simulink model "traslacion_carro"  (R2019a)
settings: Solver=VariableStepAuto  StartTime=0.0  StopTime=10.0  RelTol=1e-3
values from neighbouring files (symbols this model uses):
  b_t = 90.0    (= 90)    [parametros.m]
  b_tb = 5.0e6    (= 5000000)    [parametros.m]
  b_td_eq = ( b_td + i_t^2*b_tm ) / (r_td^2)    (= 21607.2)    [parametros.m]
  b_tw = 3.0e3    (= 3000)    [parametros.m]
  i_t = 30.0    (= 30)    [parametros.m]
  K_tw = 4.8e5    (= 480000)    [parametros.m]
  M_t = 30000    [parametros.m]
  m_td_eq = ( J_td + i_t^2*J_tm_tb ) / (r_td^2)    (= 30000)    [parametros.m]
  r_td = 0.50    (= 0.5)    [parametros.m]
  T_tb_max = 5.0e3    (= 5000)    [parametros.m]
  x_t0 = -30.0    (= -30)    [parametros.m]
  x_td0 = x_t0    (= -30)    [parametros.m]
settings Model: Creator=Facundo  LastModifiedBy=Facundo
settings DataIOCC: SaveOutput=off  SaveTime=off

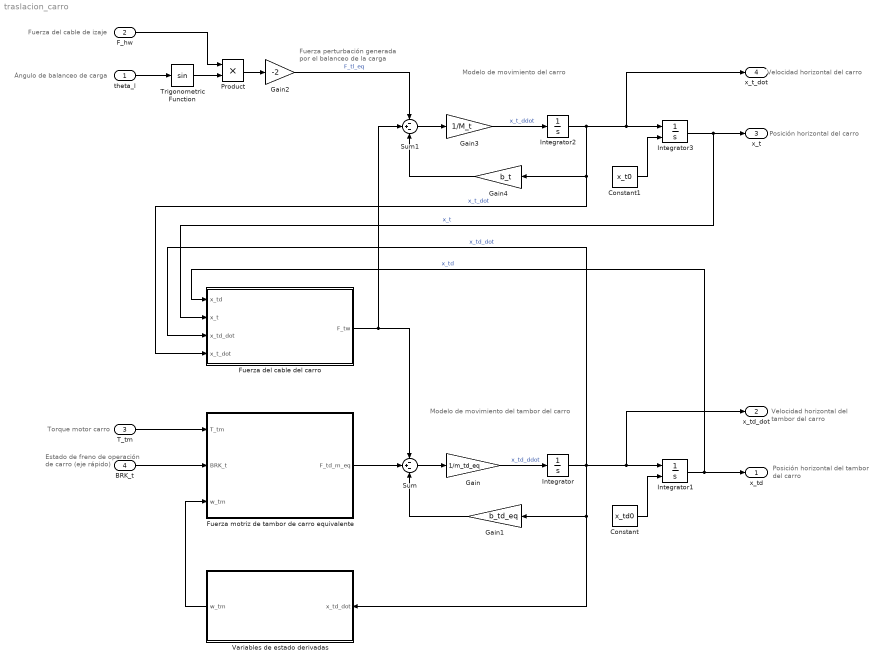
== system traslacion_carro ==
  note: Velocidad horizontal
      | del tambor del carro
  note: Velocidad horizontal del carro
  note: Modelo de movimiento del carro
  note: Fuerza perturbación generada
      | por el balanceo de la carga
  note: Posición horizontal del carro
  note: Estado de freno de
      | operación de carro
      | (eje rápido)
  note: Torque motor carro
  note: Modelo de movimiento del tambor del carro
  note: Fuerza del cable de izaje
  note: Ángulo de balanceo de carga
  note: Posición horizontal
      | del tambor del carro
  theta_l : Inport  OutDataTypeStr=double  PortDimensions=1  SampleTime=0
  F_hw : Inport  Port=2  OutDataTypeStr=double  PortDimensions=1  SampleTime=0
  T_tm : Inport  Port=3
  BRK_t : Inport  Port=4
  Constant : Constant  Value=x_td0
  Constant1 : Constant  Value=x_t0
  Fuerza del cable del carro : Subsystem
  Fuerza motriz de tambor de carro equivalente : Subsystem
  Gain : Gain  Gain=1/m_td_eq
  Gain1 : Gain  Gain=b_td_eq
  Gain2 : Gain  Gain=-2
  Gain3 : Gain  Gain=1/M_t
  Gain4 : Gain  Gain=b_t
  Integrator : Integrator
  Integrator1 : Integrator  InitialConditionSource=external
  Integrator2 : Integrator
  Integrator3 : Integrator  InitialConditionSource=external
  Product : Product
  Sum : Sum  Inputs=-+-
  Sum1 : Sum  Inputs=-+-
  Trigonometric Function : Trigonometry
  Variables de estado derivadas : Subsystem
  x_td : Outport  OutDataTypeStr=double  PortDimensions=1  SampleTime=0
  x_td_dot : Outport  Port=2  OutDataTypeStr=double  PortDimensions=1  SampleTime=0
  x_t : Outport  Port=3  OutDataTypeStr=double  PortDimensions=1  SampleTime=0
  x_t_dot : Outport  Port=4  OutDataTypeStr=double  PortDimensions=1  SampleTime=0
  wires:
  Fuerza del cable del carro/1(F_tw) -> Sum1/2, Sum/1
  Gain2/1 -> Sum1/1  "F_tl_eq"
  Integrator/1 -> Fuerza del cable del carro/3(x_td_dot), Variables de estado derivadas/1(x_td_dot), Gain1/1, x_td_dot/1, Integrator1/1  "x_td_dot"
  Sum/1 -> Gain/1
  Variables de estado derivadas/1(w_tm) -> Fuerza motriz de tambor de carro equivalente/3(w_tm)
  Constant1/1 -> Integrator3/2
  F_hw/1 -> Product/1
  BRK_t/1 -> Fuerza motriz de tambor de carro equivalente/2(BRK_t)
  Gain/1 -> Integrator/1  "x_td_ddot"
  T_tm/1 -> Fuerza motriz de tambor de carro equivalente/1(T_tm)
  Product/1 -> Gain2/1
  Gain1/1 -> Sum/3
  Trigonometric Function/1 -> Product/2
  Integrator2/1 -> Fuerza del cable del carro/4(x_t_dot), Gain4/1, x_t_dot/1, Integrator3/1  "x_t_dot"
  Gain3/1 -> Integrator2/1  "x_t_ddot"
  Integrator1/1 -> x_td/1, Fuerza del cable del carro/1(x_td)  "x_td"
  Sum1/1 -> Gain3/1
  theta_l/1 -> Trigonometric Function/1
  Gain4/1 -> Sum1/3
  Constant/1 -> Integrator1/2
  Integrator3/1 -> x_t/1, Fuerza del cable del carro/2(x_t)  "x_t"
  Fuerza motriz de tambor de carro equivalente/1(F_td_m_eq) -> Sum/2

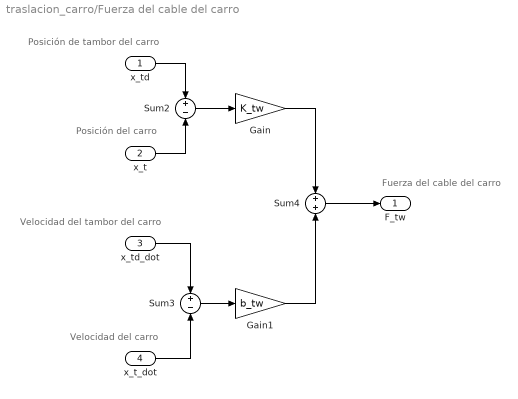
== system traslacion_carro/Fuerza del cable del carro ==
  note: Posición de tambor del carro
  note: Velocidad del tambor del carro
  note: Posición del carro
  note: Velocidad del carro
  note: Fuerza del cable del carro
  x_td : Inport
  x_t : Inport  Port=2
  x_td_dot : Inport  Port=3
  x_t_dot : Inport  Port=4
  Gain : Gain  Gain=K_tw
  Gain1 : Gain  Gain=b_tw
  Sum2 : Sum  Inputs=+-
  Sum3 : Sum  Inputs=+-
  Sum4 : Sum
  F_tw : Outport
  wires:
  x_td_dot/1 -> Sum3/1
  x_td/1 -> Sum2/1
  x_t_dot/1 -> Sum3/2
  x_t/1 -> Sum2/2
  Sum4/1 -> F_tw/1
  Gain/1 -> Sum4/1
  Sum2/1 -> Gain/1
  Gain1/1 -> Sum4/2
  Sum3/1 -> Gain1/1

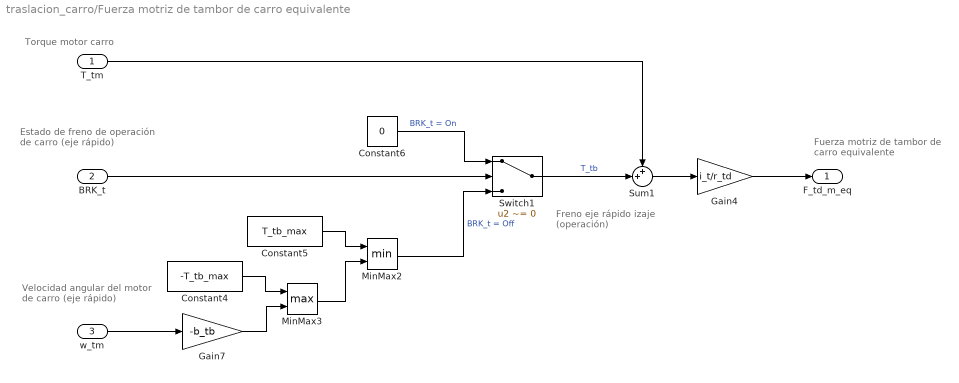
== system traslacion_carro/Fuerza motriz de tambor de carro equivalente ==
  note: Fuerza motriz de tambor
      | de carro equivalente
  note: Torque motor carro
  note: Freno eje rápido izaje
      | (operación)
  note: Estado de freno de
      | operación de carro
      | (eje rápido)
  note: Velocidad angular
      | del motor de carro
      | (eje rápido)
  T_tm : Inport
  BRK_t : Inport  Port=2  OutDataTypeStr=boolean
  w_tm : Inport  Port=3
  Constant4 : Constant  Value=-T_tb_max
  Constant5 : Constant  Value=T_tb_max
  Constant6 : Constant  Value=0
  Gain4 : Gain  Gain=i_t/r_td
  Gain7 : Gain  Gain=-b_tb
  MinMax2 : MinMax  Inputs=2
  MinMax3 : MinMax  Function=max  Inputs=2
  Sum1 : Sum  Inputs=++|
  Switch1 : Switch  Criteria=u2 ~= 0
  F_td_m_eq : Outport
  wires:
  MinMax3/1 -> MinMax2/2
  MinMax2/1 -> Switch1/3  "BRK_t = Off"
  Constant4/1 -> MinMax3/1
  T_tm/1 -> Sum1/1
  w_tm/1 -> Gain7/1
  Constant5/1 -> MinMax2/1
  Gain7/1 -> MinMax3/2
  BRK_t/1 -> Switch1/2
  Constant6/1 -> Switch1/1  "BRK_t = On"
  Sum1/1 -> Gain4/1
  Switch1/1 -> Sum1/2  "T_tb"
  Gain4/1 -> F_td_m_eq/1

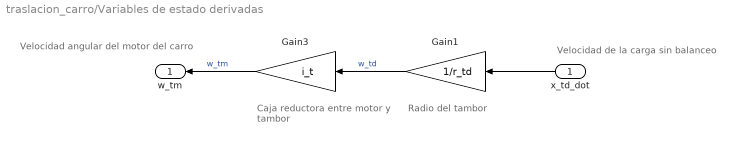
== system traslacion_carro/Variables de estado derivadas ==
  note: Radio del tambor
  note: Caja reductora
      | entre motor y tambor
  note: Velocidad angular del motor del carro
  note: Velocidad de la carga sin balanceo
  x_td_dot : Inport
  Gain1 : Gain  Gain=1/r_td
  Gain3 : Gain  Gain=i_t
  w_tm : Outport
  wires:
  Gain1/1 -> Gain3/1  "w_td"
  x_td_dot/1 -> Gain1/1
  Gain3/1 -> w_tm/1  "w_tm"
